simulink model "Aufgabe_5_2_4_Winkelsensor"  (R2023b)
settings: Solver=FixedStepDiscrete  StartTime=0.0  StopTime=10.0  FixedStep=0.01  RelTol=1e-3  EnableMultiTasking=on
settings Model: Creator=JCP  LastModifiedBy=JCP
settings SolverCC: AutoInsertRateTranBlk=on

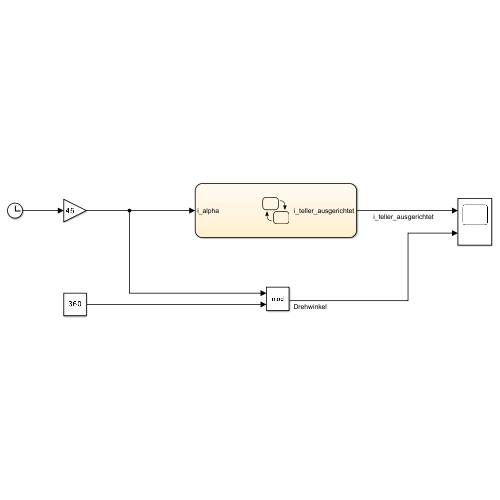
[thumbnail: Simulink's stored preview of the top-level diagram]
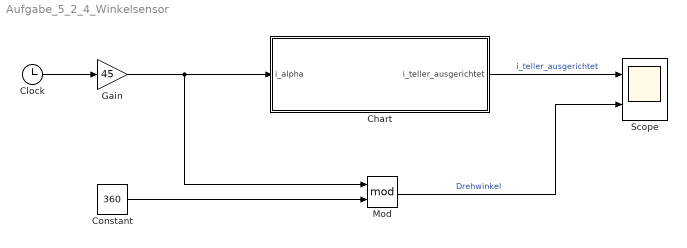
== system Aufgabe_5_2_4_Winkelsensor ==
  Chart : Stateflow chart  TreatAsAtomicUnit=on
  Clock : Clock
  Constant : Constant  Value=360
  Gain : Gain  Gain=45
  Mod : Math  Operator=mod
  Scope : Scope  NumInputPorts=2
  wires:
  Gain/1 -> Mod/1, Chart/1(i_alpha)
  Clock/1 -> Gain/1
  Chart/1(i_teller_ausgerichtet) -> Scope/1  "i_teller_ausgerichtet"
  Constant/1 -> Mod/2
  Mod/1 -> Scope/2  "Drehwinkel"

== stateflow chart Aufgabe_5_2_4_Winkelsensor/Chart ==
  state Winkelsensor
    state Ausgerichtet
      entry: i_teller_ausgerichtet = 1;
    state Nicht_ausgerichtet
      entry: i_teller_ausgerichtet = 0;
    Nicht_ausgerichtet -> Ausgerichtet : [mod(i_alpha, 90) >88 || mod(i_alpha, 90) < 2]
    (default) -> Nicht_ausgerichtet
    Ausgerichtet -> Nicht_ausgerichtet : [mod(i_alpha, 90) >= 2 && mod(i_alpha, 90) <= 88]
  data: i_alpha input; i_teller_ausgerichtet output
